simulink model "SimMonofasicoMeioLinhaComIsolador"  (R2022b)
settings: Solver=ode45  StartTime=0.0  StopTime=SimulacaoTempo  RelTol=1e-3  EnableMultiTasking=on
values from neighbouring files (symbols this model uses):
  lp = (imag(Zp)/(2*pi*f))*d    [CarregaDados.m]    (also in CarregaDados20km.m)
  m1 = n    [CurtoCircuitos.m]    (also in CurtosComparadosMonofasicos.m)
  Rmrt = ValorCurto    [CurtoCircuitos.m]
  rp = real(Zp)*d    [CarregaDados.m]    (also in CarregaDados20km.m)
libraries: spsGroundLib x6, spsSeriesRLCBranchLib x3, spsCurrentMeasurementLib x2, spsLinearTransformerLib x2, spsVoltageMeasurementLib x2, spsThreePhaseSourceLib x1, spspowerguiLib x1
settings Model: Creator=laris  LastModifiedBy=Leonardo Felipe
settings SolverCC: AlgebraicLoopSolver=TrustRegion
settings DataIOCC: LimitDataPoints=on  SaveFormat=Array  ReturnWorkspaceOutputs=off
settings OptimizationCC: LifeSpan=inf
settings DebuggingCC: UnconnectedInputMsg=warning  UnconnectedOutputMsg=warning  UnconnectedLineMsg=warning  SFUnexpectedBacktrackingDiag=warning  SFNoUnconditionalDefaultTransitionDiag=warning  SFExecutionAtInitializationDiag=none  SFMachineParentedDataDiag=warning  ArithmeticOperatorsInVariantConditions=warning
settings HardwareCC: ProdBitPerPointer=32  ProdBitPerSizeT=32  ProdBitPerPtrDiffT=32  ProdLargestAtomicFloat=None  ProdIntDivRoundTo=Undefined  ProdEndianess=Unspecified  ProdWordSize=32  ProdHWDeviceType=32-bit Generic
settings ModelReferenceCC: EnableRefExpFcnMdlSchedulingChecks=on  PropagateSignalLabelsOutOfModel=off
settings SFSimCC: SimUseLocalCustomCode=off  CustomCodeUndefinedFunction=UseInterfaceOnly
settings RTWCC: RTWUseLocalCustomCode=off  DLArmComputeVersion=19.05
settings CodeAppCC: StateflowObjectComments=on
settings GRTTargetCC: TargetLangStandard=C89/C90 (ANSI)
settings ConfigComp: CovMetricSettings=dw  CovSaveCumulativeToWorkspaceVar=on  CovSaveSingleToWorkspaceVar=on  CovExternalEMLEnable=off
settings SimscapeCC: SimscapeNormalizeSystem=off

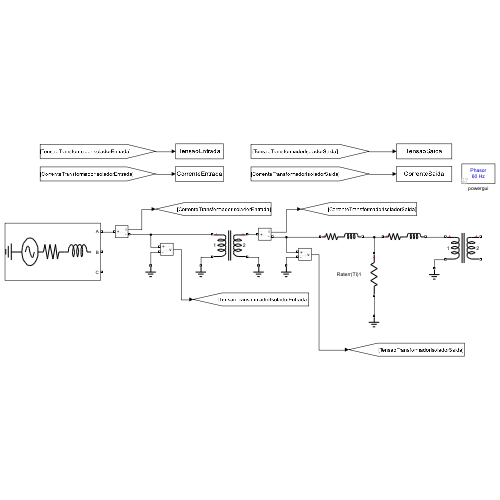
[thumbnail: Simulink's stored preview of the top-level diagram]
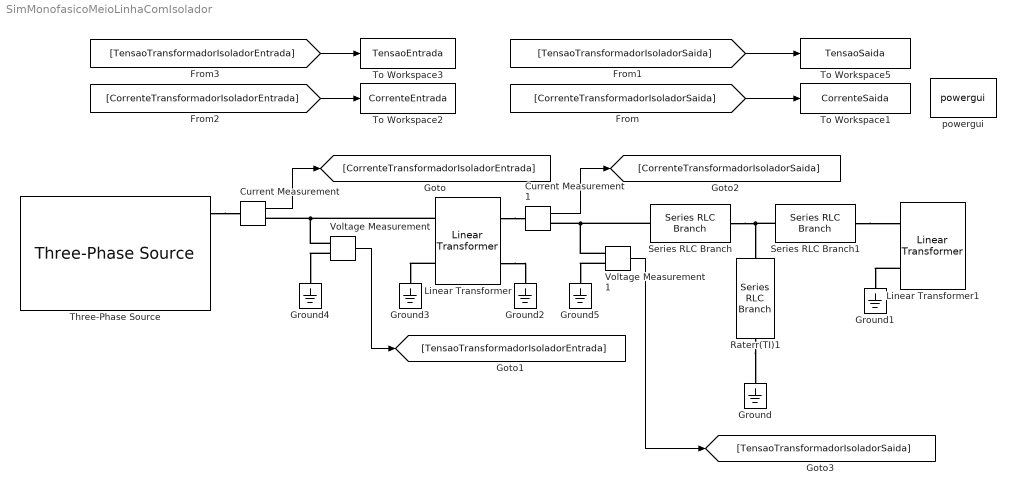
== system SimMonofasicoMeioLinhaComIsolador ==
  Current Measurement : spsCurrentMeasurementLib/Current Measurement  PhasorSimulation=on  OutputType=Complex  PSBequivalent=0
  Current Measurement1 : spsCurrentMeasurementLib/Current Measurement  PhasorSimulation=on  OutputType=Complex  PSBequivalent=0
  Ground{,1..5} (6 alike) : spsGroundLib/Ground  LConnTagsString=a
  Linear Transformer : spsLinearTransformerLib/Linear Transformer  UNITS=pu  NominalPower=[25e3 60]  winding1=[13800 0.004 0.023]  winding2=[13800/sqrt(3) 0.004 0.023]  ThreeWindings=off  winding3=[ 315e3 0.002 0.08 ]  RmLm=[ 500 500 ]  Measurements=None  DataType=off
  Linear Transformer1 : spsLinearTransformerLib/Linear Transformer  UNITS=pu  NominalPower=[25e3 60]  winding1=[13800 0.0048118 0.018511]  winding2=[380 0.0048119 0.018511]  ThreeWindings=off  winding3=[ 315e3 0.002 0.08 ]  RmLm=[ 500 500 ]  Measurements=None  DataType=off
  Raterr(TI)1 : spsSeriesRLCBranchLib/Series RLC Branch  LConnTagsString=__new0  RConnTagsString=__new0  BranchType=R  Resistance=Rmrt  Inductance=0  SetiL0=off  InitialCurrent=0  Capacitance=1e-6  Setx0=off  InitialVoltage=0  Measurements=None
  Series RLC Branch : spsSeriesRLCBranchLib/Series RLC Branch  LConnTagsString=__new0  RConnTagsString=__new0  BranchType=RL  Resistance=rp * (m1)  Inductance=lp * (m1)  SetiL0=off  InitialCurrent=0  Capacitance=0  Setx0=off  InitialVoltage=0  Measurements=None
  Series RLC Branch1 : spsSeriesRLCBranchLib/Series RLC Branch  LConnTagsString=__new0  RConnTagsString=__new0  BranchType=RL  Resistance=rp * (1-m1)  Inductance=lp * (1-m1)  SetiL0=off  InitialCurrent=0  Capacitance=0  Setx0=off  InitialVoltage=0  Measurements=None
  Three-Phase Source : spsThreePhaseSourceLib/Three-Phase Source  InternalConnection=Yg  VoltagePhases=off  Voltage=13.8e3  PhaseAngle=0  Voltage_phases=[25e3 25e3 25e3]/sqrt(3)  PhaseAngles_phases=[0 -120 +120]  Frequency=60  NonIdealSource=on  SpecifyImpedance=on  Resistance=0.8929  Inductance=16.58e-3  ShortCircuitLevel=7.2e6  BaseVoltage=13.8e3  XRratio=7  BusType=swing  Pref=10e3  Qref=0  Prefabc=[10e3, 10e3, 10e3]  Qrefabc=[0, 0, 0]  Qmin=-inf  Qmax=inf
  To Workspace1 : ToWorkspace  VariableName=CorrenteSaida  SampleTime=-1
      settings: MaxDataPoints=1
  To Workspace2 : ToWorkspace  VariableName=CorrenteEntrada  SampleTime=-1
      settings: MaxDataPoints=1
  To Workspace3 : ToWorkspace  VariableName=TensaoEntrada  SampleTime=-1
      settings: MaxDataPoints=1
  To Workspace5 : ToWorkspace  VariableName=TensaoSaida  SampleTime=-1
      settings: MaxDataPoints=1
  Voltage Measurement : spsVoltageMeasurementLib/Voltage Measurement  PhasorSimulation=on  OutputType=Complex  PSBequivalent=0
  Voltage Measurement1 : spsVoltageMeasurementLib/Voltage Measurement  PhasorSimulation=on  OutputType=Complex  PSBequivalent=0
  powergui : spspowerguiLib/powergui  Priority=1  SimulationMode=Phasor  SampleTime=50e-9  frequency=60  Iterations=50  frequencyindice=60  Pbase=100e6  ErrMax=1e-4  UnitsV=kV  UnitsW=MW  buscounter=0  FunctionMessages=off  echomessages=off  EnableUseOfTLC=off  CurrentSourceSwitches=off  DisableSnubberDevices=off  DisableRonSwitches=off  DisableVfSwitches=off  DisplayEquations=off  AutomaticDiscreteSolvers=off  SolverType=Tustin/Backward Euler (TBE)  Interpol=off  ExternalGateDelay=off  methode=off  Ts=100  x0status=blocks  SPID=on  SwTol=0  HookPort=off  NonlinearTolerance=1e-4  nMaxIteration=100  ContinueOnMaxIteration=off  RestoreLinks=warning  ResistiveCurrentMeasurement=off  Frange=[0:2:500]  Ylog=off  Xlog=on  ShowGrid=off  save=off  variable=ZData  structure=0  ZoomFFT=off  StartTime=0.0  cycles=1  DisplayStyle=1  fundamental=60  FreqAxis=off  MaxFrequency=1000  frequencyindicesteady=1  RmsSteady=1  display=off
  wires:
  [CorrenteTransformadorIsoladorSaida] -> To Workspace1/1
  [TensaoTransformadorIsoladorSaida] -> To Workspace5/1
  [CorrenteTransformadorIsoladorEntrada] -> To Workspace2/1
  [TensaoTransformadorIsoladorEntrada] -> To Workspace3/1
  Current Measurement/1 -> [CorrenteTransformadorIsoladorEntrada]
  Voltage Measurement/1 -> [TensaoTransformadorIsoladorEntrada]
  Voltage Measurement1/1 -> [TensaoTransformadorIsoladorSaida]
  Current Measurement1/1 -> [CorrenteTransformadorIsoladorSaida]
  connections:
  Raterr(TI)1/RConn1 -- Ground/LConn1
  Three-Phase Source/RConn1 -- Current Measurement/LConn1
  Voltage Measurement/LConn1 -- Linear Transformer/LConn1 -- Current Measurement/RConn1
  Voltage Measurement1/LConn1 -- Series RLC Branch/LConn1 -- Current Measurement1/RConn1
  Voltage Measurement/LConn2 -- Ground4/LConn1
  Voltage Measurement1/LConn2 -- Ground5/LConn1
  Linear Transformer/RConn1 -- Current Measurement1/LConn1
  Linear Transformer/RConn2 -- Ground2/LConn1
  Linear Transformer/LConn2 -- Ground3/LConn1
  Linear Transformer1/LConn2 -- Ground1/LConn1
  Series RLC Branch/RConn1 -- Series RLC Branch1/LConn1 -- Raterr(TI)1/LConn1
  Series RLC Branch1/RConn1 -- Linear Transformer1/LConn1
